simulink model "population"  (R2018a)
settings: Solver=VariableStepAuto  StartTime=0.0  StopTime=10.0  RelTol=1e-3
values from neighbouring files (symbols this model uses):
  a1 = 1.4    [lab1.m]    (also in populationError.m)
  a2 = a2_ideal    [lab1.m]    (also in populationError.m = Vin(2))
  d1 = 3.1    [lab1.m]    (also in populationError.m)
  d2 = -1.5    [lab1.m]    (also in populationError.m)
  N1 = 4    [lab1.m]    (also in populationError.m)
  N2 = N2_ideal    [lab1.m]    (also in populationError.m = Vin(1))
settings Model: PacingRate=100  Creator=root  LastModifiedBy=root

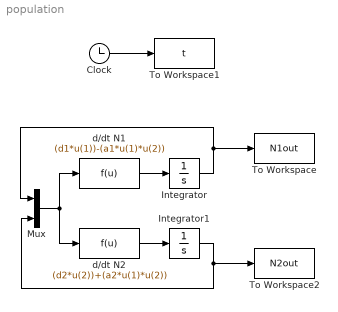
== system population ==
  Clock : Clock
  Integrator : Integrator  InitialCondition=N1
  Integrator1 : Integrator  InitialCondition=N2
  Mux : Mux  Inputs=2
  To Workspace : ToWorkspace  VariableName=N1out  SampleTime=-1
  To Workspace1 : ToWorkspace  VariableName=t  SampleTime=-1
  To Workspace2 : ToWorkspace  VariableName=N2out  SampleTime=-1
  d/dt N1 : Fcn  Expr=(d1*u(1))-(a1*u(1)*u(2))
  d/dt N2 : Fcn  Expr=(d2*u(2))+(a2*u(1)*u(2))
  wires:
  Clock/1 -> To Workspace1/1
  d/dt N1/1 -> Integrator/1
  d/dt N2/1 -> Integrator1/1
  Integrator/1 -> To Workspace/1, Mux/1
  Integrator1/1 -> To Workspace2/1, Mux/2
  Mux/1 -> d/dt N2/1, d/dt N1/1
